simulink model "Project1_Final_Option1"  (R2023b)
settings: Solver=VariableStepAuto  StartTime=0.0  StopTime=10.0  RelTol=1e-3
values from neighbouring files (symbols this model uses):
  A = A_a(2)    [Project1.m]    (also in Project1_and_graphing.m; Project1_and_graphing_plz_check.m; Project1_week1.m = 4; Project1_week2.m = [0, 100])
  b = b_a(q)    [Project1.m]    (also in Project1_and_graphing.m; Project1_and_graphing_plz_check.m; Project1_week1.m = 1; Project1_week2.m = [10, 0.1])
  freq = freq_a(p)    [Project1.m]    (also in Project1_and_graphing.m; Project1_and_graphing_plz_check.m)
  J = J_a(r)    [Project1.m]    (also in Project1_and_graphing.m; Project1_and_graphing_plz_check.m; Project1_week1.m = 1; Project1_week2.m = [100, 0.01])
  sin_check = sin_check_a(k)    [Project1.m]    (also in Project1_and_graphing.m; Project1_and_graphing_plz_check.m)
settings Model: Creator=vince  LastModifiedBy=vince

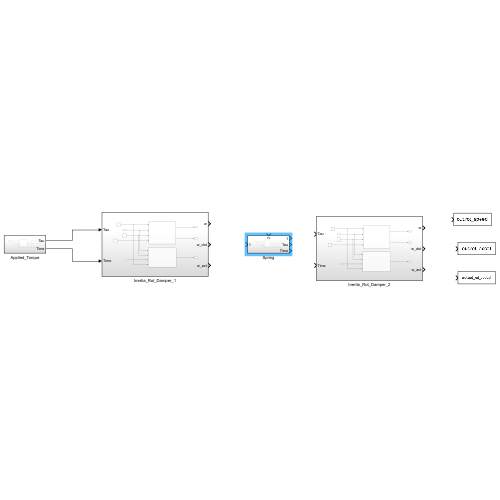
[thumbnail: Simulink's stored preview of the top-level diagram]
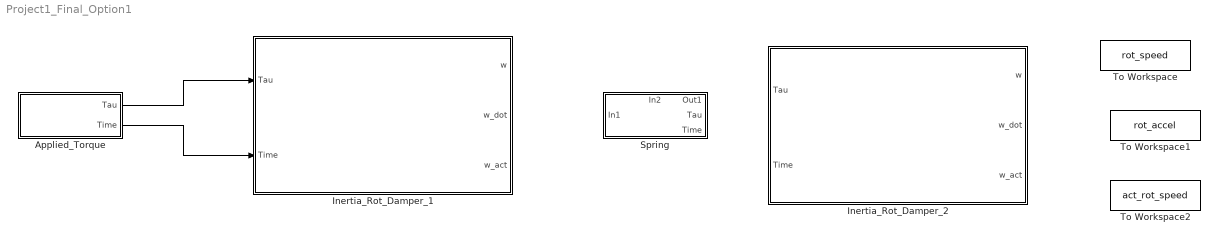
== system Project1_Final_Option1 ==
  Applied_Torque : Subsystem
  Inertia_Rot_Damper_1 : Subsystem
  Inertia_Rot_Damper_2 : Subsystem
  Spring : Subsystem
      settings: PortSchema="{\"entries\":[{\"content\":{\"sides\":[{\"content\":{\"connectorIds\":[\"In1\"]},\"type\":\"ConnectorPlacement.EquallySpacedRectSide\",\"uuid\":\"d427bc6d-98f2-4b90-b7f5-90437b246635\"},{\"content\":{\"connectorIds\":[\"Out1\",\"Out2\",\"Out3\"],\"side\":\"RIGHT\"},\"type\":\"ConnectorPlacement.EquallySpacedRectSide\",\"uuid\":\"017f07a1-a239-4d95-ace3-6c10701ac7e6\"},{\"content\":{\"connectorIds\":[\"In2\"],\"side\":\"TOP\"},\"type\":\"ConnectorPlacement.EquallySpacedRectSide\",\"uuid\":\"4793daa6-adb5-412a-917c-b5e23f88da3b\"}]},\"type\":\"ConnectorPlacement.EquallySpacedConnector\",\"uuid\":\"0390f28f-9908-474a-9e12-6fed2841a6e9\"}],\"packageUris\":[\"http://schema.mathworks.com/mf0/Connector/R2020b\"],\"version\":\"1.0\"}"
  To Workspace : ToWorkspace  VariableName=rot_speed  SaveFormat=Timeseries  SampleTime=-1
  To Workspace1 : ToWorkspace  VariableName=rot_accel  SaveFormat=Timeseries  SampleTime=-1
  To Workspace2 : ToWorkspace  VariableName=act_rot_speed  SaveFormat=Timeseries  SampleTime=-1
  wires:
  Applied_Torque/1(Tau) -> Inertia_Rot_Damper_1/1(Tau)
  Applied_Torque/2(Time) -> Inertia_Rot_Damper_1/2(Time)

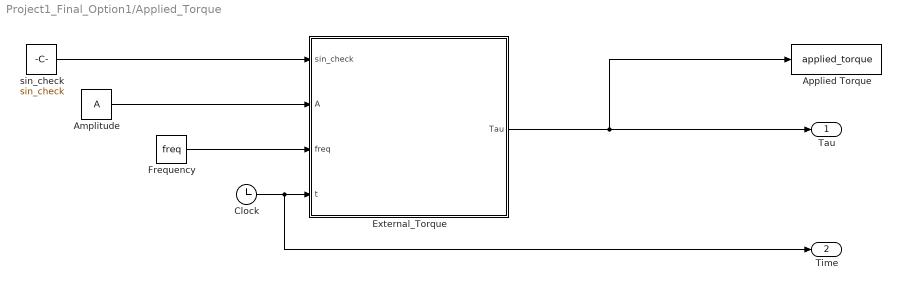
== system Project1_Final_Option1/Applied_Torque ==
  Amplitude : Constant  Value=A
  Applied Torque : ToWorkspace  VariableName=applied_torque  SaveFormat=Timeseries  SampleTime=-1
  Clock : Clock
      settings: Decimation=25
  External_Torque : MATLAB Function  TreatAsAtomicUnit=on
  Frequency : Constant  Value=freq
  sin_check : Constant  Value=sin_check
  Tau : Outport
  Time : Outport  Port=2
  wires:
  Frequency/1 -> External_Torque/3(freq)
  sin_check/1 -> External_Torque/1(sin_check)
  Amplitude/1 -> External_Torque/2(A)
  Clock/1 -> Time/1, External_Torque/4(t)
  External_Torque/1(Tau) -> Tau/1, Applied Torque/1

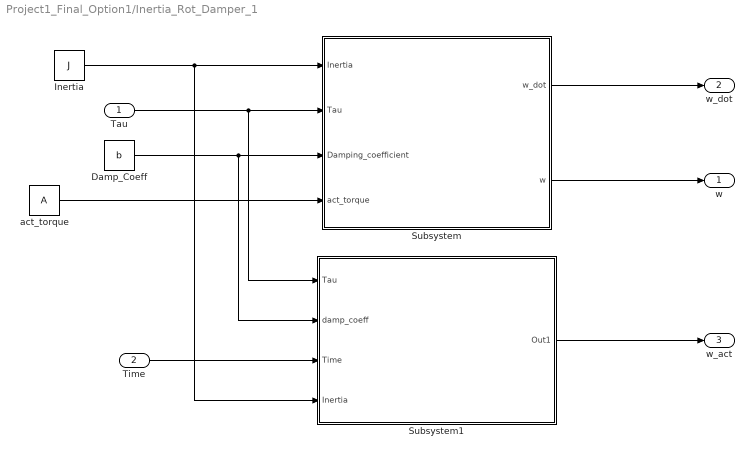
== system Project1_Final_Option1/Inertia_Rot_Damper_1 ==
  Tau : Inport
  Time : Inport  Port=2
  Damp_Coeff : Constant  Value=b
  Inertia : Constant  Value=J
  Subsystem : Subsystem
  Subsystem1 : Subsystem
  act_torque : Constant  Value=A
  w : Outport
  w_dot : Outport  Port=2
  w_act : Outport  Port=3
  wires:
  Subsystem/2(w) -> w/1
  Subsystem/1(w_dot) -> w_dot/1
  Tau/1 -> Subsystem1/1(Tau), Subsystem/2(Tau)
  Inertia/1 -> Subsystem1/4(Inertia), Subsystem/1(Inertia)
  Damp_Coeff/1 -> Subsystem1/2(damp_coeff), Subsystem/3(Damping_coefficient)
  Subsystem1/1(Out1) -> w_act/1
  Time/1 -> Subsystem1/3(Time)
  act_torque/1 -> Subsystem/4(act_torque)

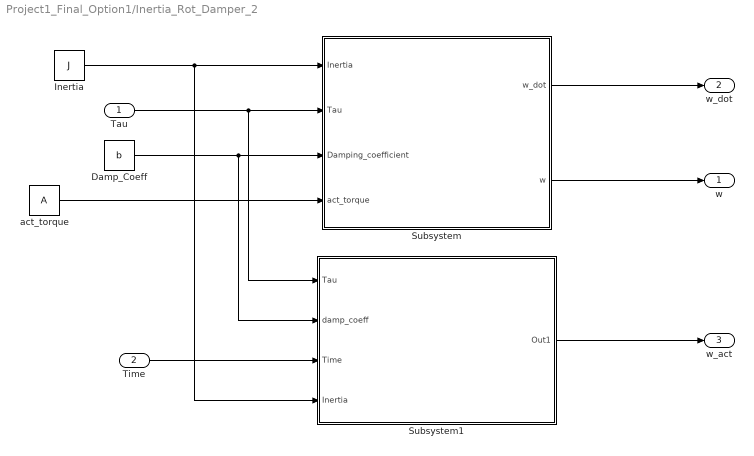
== system Project1_Final_Option1/Inertia_Rot_Damper_2 ==
  Tau : Inport
  Time : Inport  Port=2
  Damp_Coeff : Constant  Value=b
  Inertia : Constant  Value=J
  Subsystem : Subsystem
  Subsystem1 : Subsystem
  act_torque : Constant  Value=A
  w : Outport
  w_dot : Outport  Port=2
  w_act : Outport  Port=3
  wires:
  Subsystem/2(w) -> w/1
  Subsystem/1(w_dot) -> w_dot/1
  Tau/1 -> Subsystem1/1(Tau), Subsystem/2(Tau)
  Inertia/1 -> Subsystem1/4(Inertia), Subsystem/1(Inertia)
  Damp_Coeff/1 -> Subsystem1/2(damp_coeff), Subsystem/3(Damping_coefficient)
  Subsystem1/1(Out1) -> w_act/1
  Time/1 -> Subsystem1/3(Time)
  act_torque/1 -> Subsystem/4(act_torque)

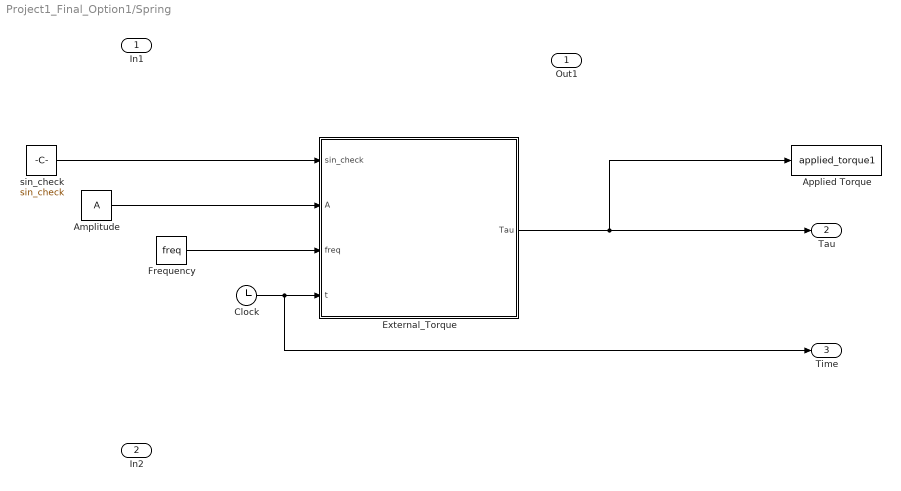
== system Project1_Final_Option1/Spring ==
  In1 : Inport
  In2 : Inport  Port=2
  Amplitude : Constant  Value=A
  Applied Torque : ToWorkspace  VariableName=applied_torque1  SaveFormat=Timeseries  SampleTime=-1
  Clock : Clock
      settings: Decimation=25
  External_Torque : MATLAB Function  TreatAsAtomicUnit=on
  Frequency : Constant  Value=freq
  sin_check : Constant  Value=sin_check
  Out1 : Outport
  Tau : Outport  Port=2
  Time : Outport  Port=3
  wires:
  External_Torque/1(Tau) -> Tau/1, Applied Torque/1
  sin_check/1 -> External_Torque/1(sin_check)
  Amplitude/1 -> External_Torque/2(A)
  Clock/1 -> Time/1, External_Torque/4(t)
  Frequency/1 -> External_Torque/3(freq)

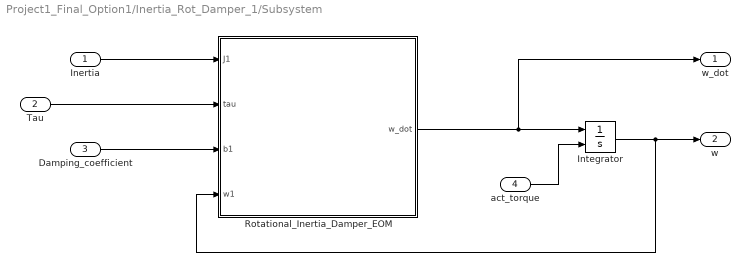
== system Project1_Final_Option1/Inertia_Rot_Damper_1/Subsystem ==
  Inertia : Inport
  Tau : Inport  Port=2
  Damping_coefficient : Inport  Port=3
  act_torque : Inport  Port=4
  Integrator : Integrator  InitialConditionSource=external
  Rotational_Inertia_Damper_EOM : MATLAB Function  TreatAsAtomicUnit=on
  w_dot : Outport
  w : Outport  Port=2
  wires:
  Integrator/1 -> Rotational_Inertia_Damper_EOM/4(w1), w/1
  Inertia/1 -> Rotational_Inertia_Damper_EOM/1(J1)
  Rotational_Inertia_Damper_EOM/1(w_dot) -> w_dot/1, Integrator/1
  Tau/1 -> Rotational_Inertia_Damper_EOM/2(tau)
  Damping_coefficient/1 -> Rotational_Inertia_Damper_EOM/3(b1)
  act_torque/1 -> Integrator/2

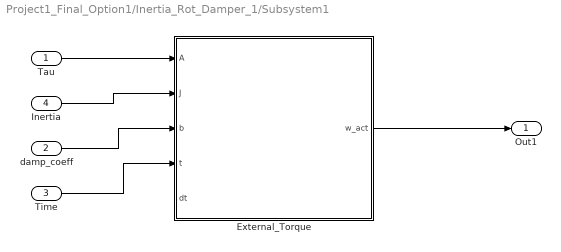
== system Project1_Final_Option1/Inertia_Rot_Damper_1/Subsystem1 ==
  Tau : Inport
  damp_coeff : Inport  Port=2
  Time : Inport  Port=3
  Inertia : Inport  Port=4
  External_Torque : MATLAB Function  TreatAsAtomicUnit=on
  Out1 : Outport
  wires:
  External_Torque/1(w_act) -> Out1/1
  Tau/1 -> External_Torque/1(A)
  Inertia/1 -> External_Torque/2(J)
  damp_coeff/1 -> External_Torque/3(b)
  Time/1 -> External_Torque/4(t)

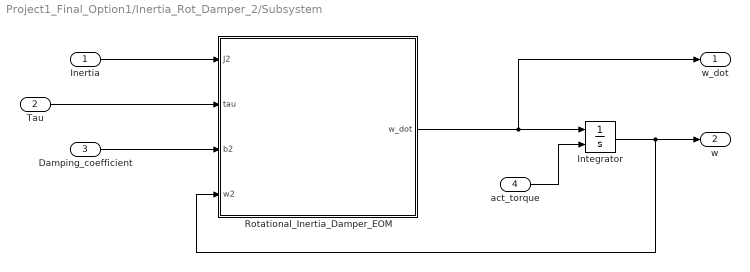
== system Project1_Final_Option1/Inertia_Rot_Damper_2/Subsystem ==
  Inertia : Inport
  Tau : Inport  Port=2
  Damping_coefficient : Inport  Port=3
  act_torque : Inport  Port=4
  Integrator : Integrator  InitialConditionSource=external
  Rotational_Inertia_Damper_EOM : MATLAB Function  TreatAsAtomicUnit=on
  w_dot : Outport
  w : Outport  Port=2
  wires:
  Integrator/1 -> Rotational_Inertia_Damper_EOM/4(w2), w/1
  Inertia/1 -> Rotational_Inertia_Damper_EOM/1(J2)
  Rotational_Inertia_Damper_EOM/1(w_dot) -> w_dot/1, Integrator/1
  Tau/1 -> Rotational_Inertia_Damper_EOM/2(tau)
  Damping_coefficient/1 -> Rotational_Inertia_Damper_EOM/3(b2)
  act_torque/1 -> Integrator/2

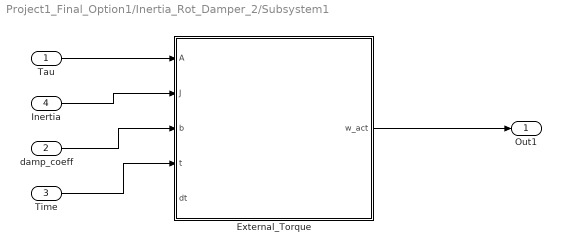
== system Project1_Final_Option1/Inertia_Rot_Damper_2/Subsystem1 ==
  Tau : Inport
  damp_coeff : Inport  Port=2
  Time : Inport  Port=3
  Inertia : Inport  Port=4
  External_Torque : MATLAB Function  TreatAsAtomicUnit=on
  Out1 : Outport
  wires:
  External_Torque/1(w_act) -> Out1/1
  Tau/1 -> External_Torque/1(A)
  Inertia/1 -> External_Torque/2(J)
  damp_coeff/1 -> External_Torque/3(b)
  Time/1 -> External_Torque/4(t)

== matlab function Project1_Final_Option1/Inertia_Rot_Damper_1/Subsystem/Rotational_Inertia_Damper_EOM ==
  data: J1 input; tau input; w_dot output; b1 input; w1 input
function w_dot = fcn(J1, tau, b1, w1)
% Recall EOM: J*w_dot = tau_applied - tau_damped
tau_damped = b1*w1;
w_dot = (1/J1)*(tau - tau_damped);
end

== matlab function Project1_Final_Option1/Applied_Torque/External_Torque ==
  data: sin_check input; Tau output; A input; freq input; t input
function Tau = fcn(sin_check, A, freq, t)

if (sin_check == 0)
    Tau = A;

else 
    Tau = A*sin(freq*t);
end

== matlab function Project1_Final_Option1/Inertia_Rot_Damper_1/Subsystem1/External_Torque ==
  data: w_act output; A input; J input; b input; t input; dt input
function w_act = fcn(A, J, b, t, dt)

w_act = zeros(size(t));

% Initial condition
w_act(1) = 0; 

% Compute angular velocity over time
for i = 2:length(t)
    % Compute angular acceleration
    alpha = (A - b * w_act(i-1)) / J;
    
    % Update angular velocity
    w_act(i) = w_act(i-1) + alpha * dt;
end

== matlab function Project1_Final_Option1/Inertia_Rot_Damper_2/Subsystem/Rotational_Inertia_Damper_EOM ==
  data: J2 input; tau input; w_dot output; b2 input; w2 input
function w_dot = fcn(J2, tau, b2, w2)
% Recall EOM: J*w_dot = tau_applied - tau_damped
tau_damped = b2*w2;
w_dot = (1/J2)*(tau - tau_damped);
end

== matlab function Project1_Final_Option1/Inertia_Rot_Damper_2/Subsystem1/External_Torque ==
  data: w_act output; A input; J input; b input; t input; dt input
function w_act = fcn(A, J, b, t, dt)

w_act = zeros(size(t));

% Initial condition
w_act(1) = 0; 

% Compute angular velocity over time
for i = 2:length(t)
    % Compute angular acceleration
    alpha = (A - b * w_act(i-1)) / J;
    
    % Update angular velocity
    w_act(i) = w_act(i-1) + alpha * dt;
end

== matlab function Project1_Final_Option1/Spring/External_Torque ==
  data: sin_check input; Tau output; A input; freq input; t input
function Tau = fcn(sin_check, A, freq, t)

if (sin_check == 0)
    Tau = A;

else 
    Tau = A*sin(freq*t);
end
